simulink model "motor_controller"  (R2015b)
settings: Solver=VariableStepAuto  StartTime=0.0  StopTime=inf  RelTol=1e-3
undefined symbols (not defined in the file or in its folder): CR, serial
libraries: instrumentlib x3, simulink x1
settings Model: Creator=andfro  LastModifiedBy=andfro

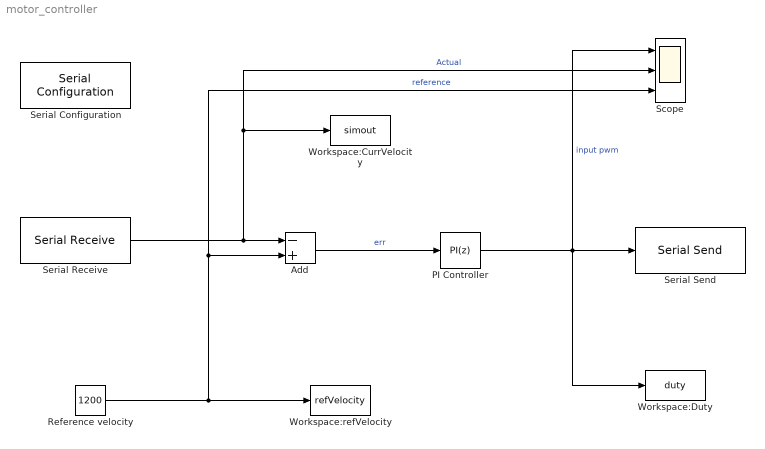
== system motor_controller ==
  " PI Controller" : simulink/Continuous/PID Controller  Controller=PI  TimeDomain=Discrete-time  SampleTime=-1  IntegratorMethod=Forward Euler  FilterMethod=Forward Euler  Form=Parallel  UseFilter=on  ControllerParametersSource=internal  P=1  I=1  D=0  N=100  InitialConditionSource=internal  InitialConditionForIntegrator=0  InitialConditionForFilter=0  ExternalReset=none  LimitOutput=on  UpperSaturationLimit=100  LowerSaturationLimit=0  LinearizeAsGain=off  AntiWindupMode=none  Kb=1  TrackingMode=off  Kt=1  PParamMin=[]  PParamMax=[]  IParamMin=[]  IParamMax=[]  DParamMin=[]  DParamMax=[]  NParamMin=[]  NParamMax=[]  KbParamMin=[]  KbParamMax=[]  KtParamMin=[]  KtParamMax=[]  POutMin=[]  POutMax=[]  IOutMin=[]  IOutMax=[]  DOutMin=[]  DOutMax=[]  NOutMin=[]  NOutMax=[]  KbOutMin=[]  KbOutMax=[]  KtOutMin=[]  KtOutMax=[]  IntegratorOutMin=[]  IntegratorOutMax=[]  FilterOutMin=[]  FilterOutMax=[]  SumOutMin=[]  SumOutMax=[]  SumOutDataTypeStr=uint8  SumI1OutMin=[]  SumI1OutMax=[]  SumI2OutMin=[]  SumI2OutMax=[]  SumI3OutMin=[]  SumI3OutMax=[]  SumDOutMin=[]  SumDOutMax=[]  SaturationOutMin=[]  SaturationOutMax=[]  IntegratorContinuousStateAttributes=''  IntegratorStateMustResolveToSignalObject=off  IntegratorRTWStateStorageClass=Auto  FilterContinuousStateAttributes=''  FilterStateMustResolveToSignalObject=off  FilterRTWStateStorageClass=Auto  DifferentiatorICPrevScaledInput=0  DifferentiatorOutMin=[]  DifferentiatorOutMax=[]
  Add : Sum  Inputs=-+
  Reference velocity : Constant  Value=1200
  Scope : Scope  NumInputPorts=3
  Serial Configuration : instrumentlib/Serial Configuration  Priority=-200000  ComPortMenu=COM26  ComPort=COM26  ObjConstructor=serial('COM26');  BaudRate=115200  DataBits=8  Parity=none  StopBits=1  FlowControl=none  Timeout=10  ByteOrder=LittleEndian
  Serial Receive : instrumentlib/Serial Receive  ComPortMenu=COM26  ComPort=COM26  ObjConstructor=serial('COM26');  Terminator=<none>  DataSize=[1 1]  DataType=uint8  EnableBlockingMode=on  ActionDataUnavailable=Output last received value  CustomValue=0  SampleTime=0.01
  Serial Send : instrumentlib/Serial Send  ComPortMenu=COM26  ComPort=COM26  ObjConstructor=serial('COM26');  Terminator=CR ('\r')  EnableBlockingMode=on
  Workspace:CurrVelocity : ToWorkspace  VariableName=simout  SaveFormat=Timeseries  SampleTime=-1
  Workspace:Duty : ToWorkspace  VariableName=duty  SaveFormat=Timeseries  SampleTime=-1
  Workspace:refVelocity : ToWorkspace  VariableName=refVelocity  SaveFormat=Timeseries  SampleTime=-1
  wires:
  Serial Receive/1 -> Scope/2, Workspace:CurrVelocity/1, Add/1  "Actual"
  Add/1 -> " PI Controller"/1  "err"
  " PI Controller"/1 -> Scope/1, Workspace:Duty/1, Serial Send/1  "input pwm"
  Reference velocity/1 -> Workspace:refVelocity/1, Scope/3, Add/2  "reference"
